simulink model "rtwdemo_autosar_multirunnables"  (Simulink 7.6)
settings: Solver=FixedStepDiscrete  StartTime=0.0  StopTime=0.025  FixedStep=0.001  MaxStep=.0001  RelTol=1e-3
undefined symbols (not defined in the file or in its folder): DiscIntNeverNeededParam
Description:
  | Modeling AUTOSAR multirunnables
CloseFcn:
  | rtwprivate ssgencode ModelCloseRequest case1_modified
settings Model: Creator=The MathWorks Inc.  ExtModeAutoUpdateStatusClock=off
settings MATStruct: SampleTime=0.001  Offset=0  Priority=[20.0]
settings DataIOCC: SaveOutput=off  SaveTime=off
settings OptimizationCC: InlineParams=on  InlineInvariantSignals=on  StateBitsets=on  DataBitsets=on  UseTempVars=on  ZeroExternalMemoryAtStartup=off  ZeroInternalMemoryAtStartup=off  NoFixptDivByZeroProtection=on  EfficientFloat2IntCast=on  EfficientMapNaN2IntZero=off  OptimizeModelRefInitCode=on  LifeSpan=1  BufferReusableBoundary=off
settings DebuggingCC: SolverPrmCheckMsg=none  SigSpecEnsureSampleTimeMsg=none  BusObjectLabelMismatch=none  StrictBusMsg=ErrorOnBusTreatedAsVector
settings HardwareCC: ProdIntDivRoundTo=Zero  ProdEndianess=LittleEndian  ProdHWDeviceType=Generic->32-bit Embedded Processor  TargetIntDivRoundTo=Zero  TargetEndianess=LittleEndian  TargetHWDeviceType=Generic->32-bit Embedded Processor
settings SFSimCC: SimParseCustomCode=off
settings RTWCC: SystemTargetFile=autosar.tlc  GenCodeOnly=on  TemplateMakefile=ert_default_tmf  Description=AUTOSAR  GenerateReport=on  RTWVerbose=off  ProcessScript=autosar_make_rtw_hook  IncludeHyperlinkInReport=on  LaunchReport=on  GenerateCodeInfo=on
settings CodeAppCC: ForceParamTrailComments=on  IgnoreCustomStorageClasses=off  IgnoreTestpoints=on  SimulinkDataObjDesc=on  CustomSymbolStrGlobalVar=rt$N$M  CustomSymbolStrType=$N$M  CustomSymbolStrFcn=$N$M$F  CustomSymbolStrMacro=$N$M  InsertBlockDesc=on
settings STFCustomTargetCC: CompOptLevelCompliant=on  IncludeMdlTerminateFcn=off  CombineOutputUpdateFcns=on  SuppressErrorStatus=on  ERTFirstTimeCompliant=on  ERTCustomFileBanners=on  SupportNonFinite=off  SupportComplex=off  SupportContinuousTime=off  SupportNonInlinedSFcns=off  CPPClassGenCompliant=on  AutosarCompliant=on  SystemTargetFile=autosar.tlc
settings ERTTargetCC: MultiwordLength=2048  ParMdlRefBuildCompliant=off  IncludeMdlTerminateFcn=off  SuppressErrorStatus=on  SupportNonFinite=off  SupportComplex=off  ModelStepFunctionPrototypeControlCompliant=off  AutosarCompliant=on  ExtModeMexFile=noextcomm  InlinedParameterPlacement=NonHierarchical  ERTCustomFileTemplate=example_file_process.tlc  ERTFilePackagingFormat=CompactWithDataFile  ConvertIfToSwitch=off
settings CustomProperty: DataType=RTWOptions_EnumType__toolbox_rtw_targets_AUTOSAR_AUTOSAR_autosar_1_1AutosarSchemaVersion  Value=3.1
settings EnumStrPairs: String=2.0

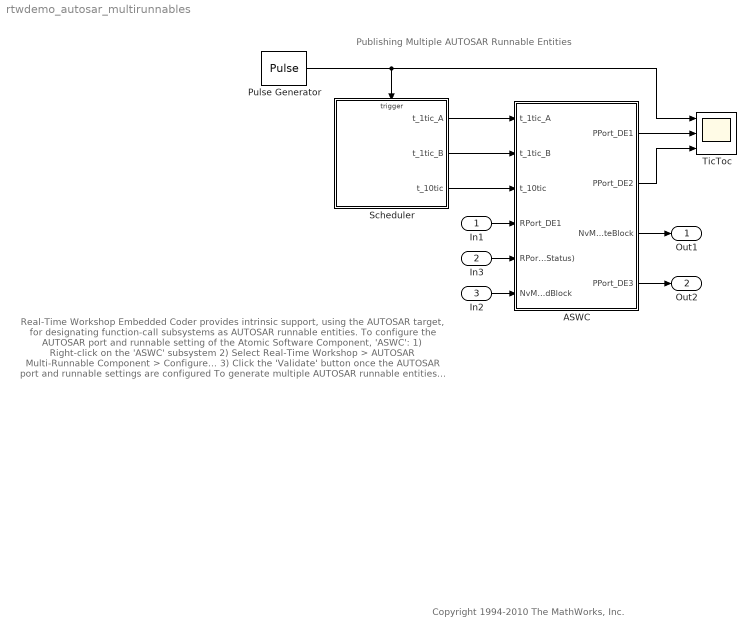
== system rtwdemo_autosar_multirunnables ==
  note: Copyright 1994-2010 The MathWorks, Inc.
  note: Publishing Multiple AUTOSAR Runnable Entities
  note: Real-Time Workshop Embedded Coder provides intrinsic support, using the AUTOSAR target,
      | for designating function-call subsystems as AUTOSAR runnable entities.
      |
      | To configure the AUTOSAR port and runnable setting of the Atomic Software Component, 'ASWC':
      |
      | 1) Right-click on the 'ASWC' subsystem
      | 2) Select Real-Time Workshop > AUTOSAR Multi-Runnable Component > Configure...
      | 3) Click the 'Validate' button once the AUTOSAR port and runnable settings are configured
      |
      | To generate multiple AUTOSAR runnable entities for a collection of function-call subsystems:
      |
      | 1) Right-click on the 'ASWC' subsystem
      | 2) Select Real-Time Workshop > AUTOSAR Multi-Runnable Component > Export Functions...
      | 3) Click the 'Build' button once the parameter dialog appears
  In1 : Inport  OutDataTypeStr=double  PortDimensions=1  SampleTime=0.001
  In3 : Inport  Port=2  OutDataTypeStr=uint8  PortDimensions=1  SampleTime=0.001
  In2 : Inport  Port=3  OutDataTypeStr=double  PortDimensions=1  SampleTime=0.001
  ASWC : Subsystem
  Pulse Generator : DiscretePulseGenerator  SampleTime=.001
  Scheduler : Stateflow chart  TreatAsAtomicUnit=on
  TicToc : Scope  NumInputPorts=3
      settings: TimeRange=0.025  YMin=0~-1~-1  YMax=1~1~1
  Out1 : Outport
  Out2 : Outport  Port=2
  wires:
  Scheduler/1(t_1tic_A) -> ASWC/1(t_1tic_A)
  Scheduler/2(t_1tic_B) -> ASWC/2(t_1tic_B)
  Pulse Generator/1 -> Scheduler/Trigger, TicToc/1
  In1/1 -> ASWC/4(RPort_DE1)
  In2/1 -> ASWC/6(NvM_ReadBlock)
  ASWC/3(NvM_WriteBlock) -> Out1/1
  ASWC/2(PPort_DE2) -> TicToc/3
  ASWC/1(PPort_DE1) -> TicToc/2
  Scheduler/3(t_10tic) -> ASWC/3(t_10tic)
  ASWC/4(PPort_DE3) -> Out2/1
  In3/1 -> ASWC/5(RPort_DE1 (ErrorStatus))

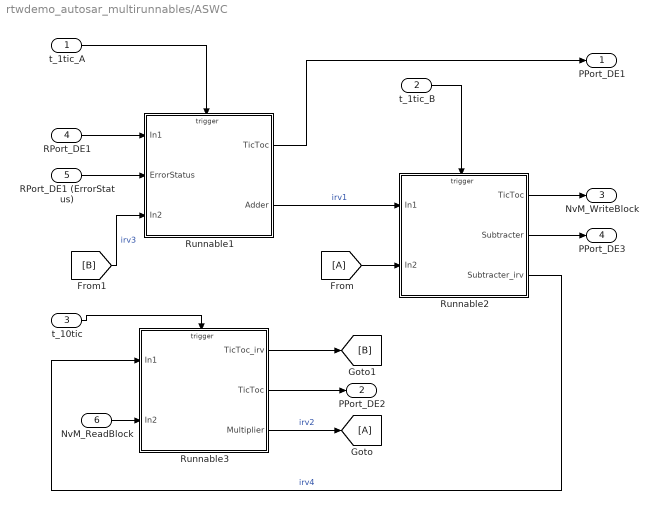
== system rtwdemo_autosar_multirunnables/ASWC ==
  t_1tic_A : Inport
  t_1tic_B : Inport  Port=2
  t_10tic : Inport  Port=3
  RPort_DE1 : Inport  Port=4
  RPort_DE1 (ErrorStatus) : Inport  Port=5
  NvM_ReadBlock : Inport  Port=6
  Runnable1 : Subsystem  TreatAsAtomicUnit=on  RTWFcnName=foo
  Runnable2 : Subsystem  TreatAsAtomicUnit=on  RTWFcnName=foo
  Runnable3 : Subsystem  TreatAsAtomicUnit=on  RTWFcnName=foo
  PPort_DE1 : Outport
  PPort_DE2 : Outport  Port=2
  NvM_WriteBlock : Outport  Port=3
  PPort_DE3 : Outport  Port=4
  wires:
  t_10tic/1 -> Runnable3/Trigger
  NvM_ReadBlock/1 -> Runnable3/2(In2)
  Runnable2/3(Subtracter_irv) -> Runnable3/1(In1)  "irv4"
  Runnable1/2(Adder) -> Runnable2/1(In1)  "irv1"
  t_1tic_A/1 -> Runnable1/Trigger
  Runnable3/2(TicToc) -> PPort_DE2/1
  Runnable2/1(TicToc) -> NvM_WriteBlock/1
  Runnable1/1(TicToc) -> PPort_DE1/1
  t_1tic_B/1 -> Runnable2/Trigger
  RPort_DE1/1 -> Runnable1/1(In1)
  Runnable2/2(Subtracter) -> PPort_DE3/1
  RPort_DE1 (ErrorStatus)/1 -> Runnable1/2(ErrorStatus)
  Runnable3/3(Multiplier) -> [A]  "irv2"
  [A] -> Runnable2/2(In2)
  Runnable3/1(TicToc_irv) -> [B]
  [B] -> Runnable1/3(In2)  "irv3"

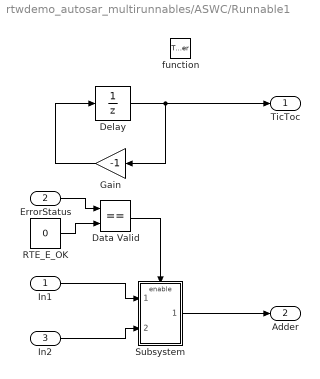
== system rtwdemo_autosar_multirunnables/ASWC/Runnable1 ==
  In1 : Inport
  ErrorStatus : Inport  Port=2
  In2 : Inport  Port=3
  function : TriggerPort  TriggerType=function-call
  Data Valid : RelationalOperator  Operator===  OutDataTypeStr=boolean
  Delay : UnitDelay  X0=1  SampleTime=-1
  Gain : Gain  Gain=-1  OutDataTypeStr=fixdt(1,8,0)
  RTE_E_OK : Constant  Value=0
  Subsystem : Subsystem
  TicToc : Outport  InitialOutput=0
  Adder : Outport  Port=2  InitialOutput=0
  wires:
  Subsystem/1(Out1) -> Adder/1
  Gain/1 -> Delay/1
  Delay/1 -> TicToc/1, Gain/1
  In1/1 -> Subsystem/1(In1)
  In2/1 -> Subsystem/2(In2)
  Data Valid/1 -> Subsystem/Enable
  ErrorStatus/1 -> Data Valid/1
  RTE_E_OK/1 -> Data Valid/2

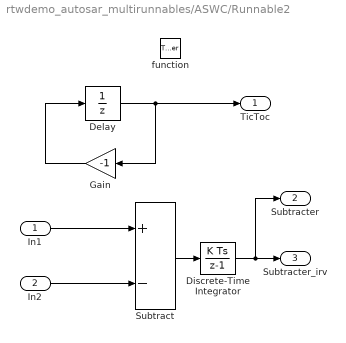
== system rtwdemo_autosar_multirunnables/ASWC/Runnable2 ==
  In1 : Inport
  In2 : Inport  Port=2
  function : TriggerPort  TriggerType=function-call
  Delay : UnitDelay  X0=1  SampleTime=-1
  Discrete-Time Integrator : DiscreteIntegrator  SampleTime=-1  ICPrevOutput=DiscIntNeverNeededParam  ICPrevScaledInput=DiscIntNeverNeededParam
  Gain : Gain  Gain=-1  OutDataTypeStr=fixdt(1,8,0)
  Subtract : Sum  Inputs=+-
  TicToc : Outport  InitialOutput=0
  Subtracter : Outport  Port=2  InitialOutput=0
  Subtracter_irv : Outport  Port=3
  wires:
  In2/1 -> Subtract/2
  In1/1 -> Subtract/1
  Delay/1 -> Gain/1, TicToc/1
  Gain/1 -> Delay/1
  Subtract/1 -> Discrete-Time Integrator/1
  Discrete-Time Integrator/1 -> Subtracter_irv/1, Subtracter/1

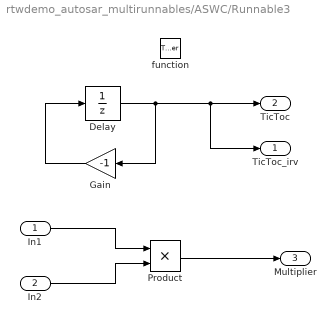
== system rtwdemo_autosar_multirunnables/ASWC/Runnable3 ==
  In1 : Inport  OutDataTypeStr=double
  In2 : Inport  Port=2
  function : TriggerPort  TriggerType=function-call
  Delay : UnitDelay  X0=1  SampleTime=-1
  Gain : Gain  Gain=-1  OutDataTypeStr=fixdt(1,8,0)
  Product : Product  Inputs=**  OutDataTypeStr=Inherit: Same as first input
  TicToc_irv : Outport
  TicToc : Outport  Port=2  InitialOutput=0
  Multiplier : Outport  Port=3  InitialOutput=0
  wires:
  In2/1 -> Product/2
  In1/1 -> Product/1
  Delay/1 -> Gain/1, TicToc/1, TicToc_irv/1
  Gain/1 -> Delay/1
  Product/1 -> Multiplier/1

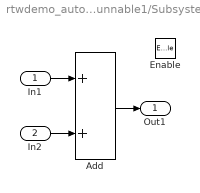
== system rtwdemo_autosar_multirunnables/ASWC/Runnable1/Subsystem ==
  In1 : Inport
  In2 : Inport  Port=2
  Enable : EnablePort
  Add : Sum
  Out1 : Outport
  wires:
  In1/1 -> Add/1
  Add/1 -> Out1/1
  In2/1 -> Add/2

== stateflow chart Scheduler ==
  settings: executeAtInitialization=1
  state OneTic [parallel]
    on every(1,tic):
    t_1tic_B; t_1tic_A;
    settings: executionOrder=1
  state TenTic [parallel]
    on every(10,tic): t_10tic;
    settings: executionOrder=2
  events: tic input EITHER_EDGE_EVENT; t_1tic_A output FUNCTION_CALL_EVENT; t_1tic_B output FUNCTION_CALL_EVENT; t_10tic output FUNCTION_CALL_EVENT
